simulink model "model6_yes"  (R2022a)
settings: Solver=FixedStepAuto  StartTime=0.0  StopTime=5  FixedStep=1e-5  RelTol=1e-3
model workspace (MAT data in the model file):
  b1 = 150
  b2 = 1500
  downSpringHeight = 10
  g = 9.81
  groundHeight = 100
  k1 = 7000
  k2 = 10000000
  m1 = 3.6
  m1IniHeight = 0
  m2 = 3.6
  m3 = 3.6
  upSpringHeight = 10
undefined symbols (not defined in the file or in its folder): DiscIntNeverNeededParam
settings Model: Creator=Tsing  LastModifiedBy=Tsing

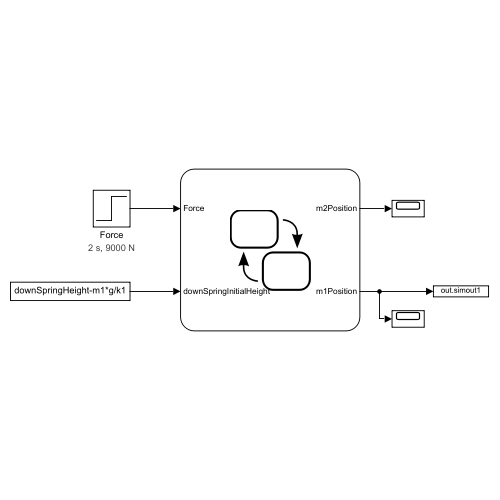
[thumbnail: Simulink's stored preview of the top-level diagram]
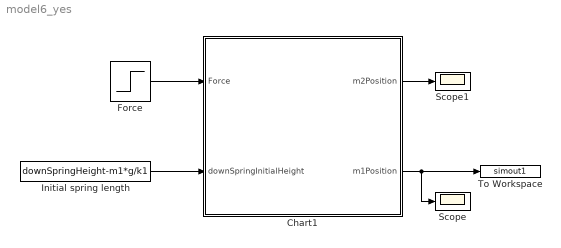
== system model6_yes ==
  Chart1 : Stateflow chart  TreatAsAtomicUnit=on
  Force : Step  Time=2  After=9000  SampleTime=0
      settings: AttributesFormatString=%<Time> s, %<After> N
  Initial spring length : Constant  Value=downSpringHeight-m1*g/k1
  Scope : Scope
  Scope1 : Scope
  To Workspace : ToWorkspace  VariableName=simout1  SaveFormat=Timeseries  SampleTime=-1
  wires:
  Force/1 -> Chart1/1(Force)
  Chart1/2(m1Position) -> To Workspace/1, Scope/1
  Initial spring length/1 -> Chart1/2(downSpringInitialHeight)
  Chart1/1(m2Position) -> Scope1/1

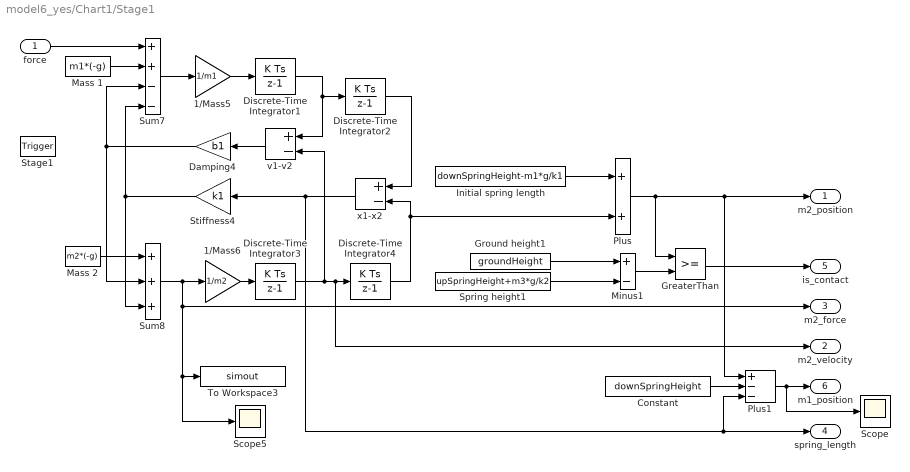
== system model6_yes/Chart1/Stage1 ==
  force : Inport  OutMin=1  OutMax=1  OutDataTypeStr=double  PortDimensions=1
  Stage1 : TriggerPort  TriggerType=function-call  VariantControl=(inherit)
      settings: CopyFcn=Stateflow.SLINSF.SimulinkMan.removeBlockPreDeleteFcn  PreDeleteFcn=Stateflow.SLINSF.SimulinkMan.unsafePredeleteFcn
  1/Mass5 : Gain  Gain=1/m1  SaturateOnIntegerOverflow=on  OutDataTypeStr=Inherit: Same as input  ParamDataTypeStr=Inherit: Same as input
  1/Mass6 : Gain  Gain=1/m2  SaturateOnIntegerOverflow=on  OutDataTypeStr=Inherit: Same as input  ParamDataTypeStr=Inherit: Same as input
  Constant : Constant  Value=downSpringHeight
  Damping4 : Gain  Gain=b1  SaturateOnIntegerOverflow=on  OutDataTypeStr=Inherit: Same as input  ParamDataTypeStr=Inherit: Same as input
  Discrete-Time Integrator1 : DiscreteIntegrator  InitialCondition=0.0  SampleTime=-1  ICPrevOutput=DiscIntNeverNeededParam  ICPrevScaledInput=DiscIntNeverNeededParam
  Discrete-Time Integrator2 : DiscreteIntegrator  InitialCondition=-m1*g/k1  SampleTime=-1  ICPrevOutput=DiscIntNeverNeededParam  ICPrevScaledInput=DiscIntNeverNeededParam
      settings: AttributesFormatString=x0 = %<InitialCondition> m
  Discrete-Time Integrator3 : DiscreteIntegrator  InitialCondition=0.0  SampleTime=-1  ICPrevOutput=DiscIntNeverNeededParam  ICPrevScaledInput=DiscIntNeverNeededParam
  Discrete-Time Integrator4 : DiscreteIntegrator  InitialCondition=0.0  SampleTime=-1  ICPrevOutput=DiscIntNeverNeededParam  ICPrevScaledInput=DiscIntNeverNeededParam
  GreaterThan : RelationalOperator  OutDataTypeStr=boolean  RndMeth=Simplest  InputSameDT=off
  Ground height1 : Constant  Value=groundHeight
  Initial spring length : Constant  Value=downSpringHeight-m1*g/k1
  Mass 1 : Constant  Value=m1*(-g)
  Mass 2 : Constant  Value=m2*(-g)
  Minus1 : Sum  Inputs=+-
  Plus : Sum
  Plus1 : Sum  Inputs=+--
  Scope : Scope
  Scope5 : Scope
  Spring height1 : Constant  Value=upSpringHeight+m3*g/k2
  Stiffness4 : Gain  Gain=k1  SaturateOnIntegerOverflow=on  OutDataTypeStr=Inherit: Same as input  ParamDataTypeStr=Inherit: Same as input
  Sum7 : Sum  Inputs=++--  InputSameDT=on  SaturateOnIntegerOverflow=on  OutDataTypeStr=Inherit: Same as first input
  Sum8 : Sum  Inputs=+++  InputSameDT=on  SaturateOnIntegerOverflow=on  OutDataTypeStr=Inherit: Same as first input
  To Workspace3 : ToWorkspace  VariableName=simout  SaveFormat=Timeseries  SampleTime=-1
  v1-v2 : Sum  Inputs=+-
  x1-x2 : Sum  Inputs=+-
  m2_position : Outport
  m2_velocity : Outport  Port=2
  m2_force : Outport  Port=3
  spring_length : Outport  Port=4
  is_contact : Outport  Port=5
  m1_position : Outport  Port=6
  wires:
  v1-v2/1 -> Damping4/1
  Sum8/1 -> Scope5/1, To Workspace3/1, m2_force/1, 1/Mass6/1
  Mass 2/1 -> Sum8/1
  force/1 -> Sum7/1
  Discrete-Time Integrator1/1 -> v1-v2/1, Discrete-Time Integrator2/1
  1/Mass6/1 -> Discrete-Time Integrator3/1
  Discrete-Time Integrator3/1 -> m2_velocity/1, Discrete-Time Integrator4/1, v1-v2/2
  Initial spring length/1 -> Plus/1
  Discrete-Time Integrator2/1 -> x1-x2/1
  Discrete-Time Integrator4/1 -> x1-x2/2, Plus/2
  x1-x2/1 -> Plus1/3, spring_length/1, Stiffness4/1
  Mass 1/1 -> Sum7/2
  1/Mass5/1 -> Discrete-Time Integrator1/1
  Plus/1 -> Plus1/1, m2_position/1, GreaterThan/1
  Stiffness4/1 -> Sum7/4, Sum8/3
  Sum7/1 -> 1/Mass5/1
  Damping4/1 -> Sum7/3, Sum8/2
  Ground height1/1 -> Minus1/1
  Spring height1/1 -> Minus1/2
  Minus1/1 -> GreaterThan/2
  GreaterThan/1 -> is_contact/1
  Plus1/1 -> Scope/1, m1_position/1
  Constant/1 -> Plus1/2

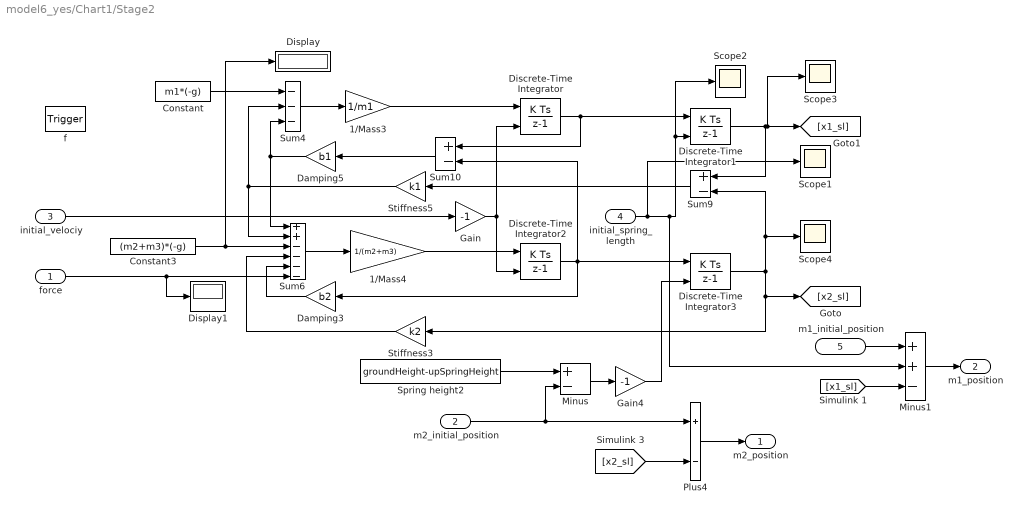
== system model6_yes/Chart1/Stage2 ==
  force : Inport  OutMin=1  OutMax=1  OutDataTypeStr=double  PortDimensions=1
  m2_initial_position : Inport  Port=2  OutMin=1  OutMax=1  OutDataTypeStr=double  PortDimensions=1
  initial_velociy : Inport  Port=3  OutMin=1  OutMax=1  OutDataTypeStr=double  PortDimensions=1
  initial_spring_length : Inport  Port=4  OutMin=1  OutMax=1  OutDataTypeStr=double  PortDimensions=1
  m1_initial_position : Inport  Port=5  OutMin=1  OutMax=1  OutDataTypeStr=double  PortDimensions=1
  f : TriggerPort  TriggerType=function-call  VariantControl=(inherit)
      settings: CopyFcn=Stateflow.SLINSF.SimulinkMan.removeBlockPreDeleteFcn  PreDeleteFcn=Stateflow.SLINSF.SimulinkMan.unsafePredeleteFcn
  1/Mass3 : Gain  Gain=1/m1  SaturateOnIntegerOverflow=on  OutDataTypeStr=Inherit: Same as input  ParamDataTypeStr=Inherit: Same as input
  1/Mass4 : Gain  Gain=1/(m2+m3)  SaturateOnIntegerOverflow=on  OutDataTypeStr=Inherit: Same as input  ParamDataTypeStr=Inherit: Same as input
  Constant : Constant  Value=m1*(-g)  SampleTime=-1
  Constant3 : Constant  Value=(m2+m3)*(-g)  SampleTime=-1
  Damping3 : Gain  Gain=b2  SaturateOnIntegerOverflow=on  OutDataTypeStr=Inherit: Same as input  ParamDataTypeStr=Inherit: Same as input
  Damping5 : Gain  Gain=b1  SaturateOnIntegerOverflow=on  OutDataTypeStr=Inherit: Same as input  ParamDataTypeStr=Inherit: Same as input
  Discrete-Time Integrator{,1..3} (4 alike) : DiscreteIntegrator  InitialConditionSource=external  SampleTime=-1  ICPrevOutput=DiscIntNeverNeededParam  ICPrevScaledInput=DiscIntNeverNeededParam
  Display : Display
  Display1 : Display
  Gain : Gain  Gain=-1
  Gain4 : Gain  Gain=-1
  Minus : Sum  Inputs=+-
  Minus1 : Sum  Inputs=++-
  Plus4 : Sum  Inputs=+-
  Scope{1..4} (4 alike) : Scope
  Spring height2 : Constant  Value=groundHeight-upSpringHeight  SampleTime=-1
  Stiffness3 : Gain  Gain=k2  SaturateOnIntegerOverflow=on  OutDataTypeStr=Inherit: Same as input  ParamDataTypeStr=Inherit: Same as input
  Stiffness5 : Gain  Gain=k1  SaturateOnIntegerOverflow=on  OutDataTypeStr=Inherit: Same as input  ParamDataTypeStr=Inherit: Same as input
  Sum10 : Sum  Inputs=+-  InputSameDT=on  SaturateOnIntegerOverflow=on  OutDataTypeStr=Inherit: Same as first input
  Sum4 : Sum  Inputs=---  InputSameDT=on  SaturateOnIntegerOverflow=on  OutDataTypeStr=Inherit: Same as first input
  Sum6 : Sum  Inputs=++----  InputSameDT=on  SaturateOnIntegerOverflow=on  OutDataTypeStr=Inherit: Same as first input
  Sum9 : Sum  Inputs=+-  InputSameDT=on  SaturateOnIntegerOverflow=on  OutDataTypeStr=Inherit: Same as first input
  m2_position : Outport
  m1_position : Outport  Port=2
  wires:
  Constant/1 -> Sum4/1
  Discrete-Time Integrator3/1 -> Scope4/1, Sum9/2, Stiffness3/1, [x2_sl]
  Damping3/1 -> Sum6/5
  Gain4/1 -> Discrete-Time Integrator3/2
  Sum4/1 -> 1/Mass3/1
  Sum6/1 -> 1/Mass4/1
  Gain/1 -> Discrete-Time Integrator2/2, Discrete-Time Integrator/2
  Plus4/1 -> m2_position/1
  m2_initial_position/1 -> Minus/2, Plus4/1
  Sum9/1 -> Stiffness5/1
  Stiffness5/1 -> Sum6/2, Sum4/2
  1/Mass4/1 -> Discrete-Time Integrator2/1
  Discrete-Time Integrator2/1 -> Sum10/2, Discrete-Time Integrator3/1, Damping3/1
  [x2_sl] -> Plus4/2
  Stiffness3/1 -> Sum6/4
  Damping5/1 -> Sum4/3, Sum6/1
  force/1 -> Sum6/6, Display1/1
  Constant3/1 -> Display/1, Sum6/3
  initial_velociy/1 -> Gain/1
  Sum10/1 -> Damping5/1
  Discrete-Time Integrator/1 -> Discrete-Time Integrator1/1, Sum10/1
  Discrete-Time Integrator1/1 -> Scope3/1, [x1_sl], Sum9/1
  1/Mass3/1 -> Discrete-Time Integrator/1
  Minus/1 -> Gain4/1
  Spring height2/1 -> Minus/1
  initial_spring_length/1 -> Scope1/1, Minus1/2, Scope2/1, Discrete-Time Integrator1/2
  Minus1/1 -> m1_position/1
  m1_initial_position/1 -> Minus1/1
  [x1_sl] -> Minus1/3

== stateflow chart model6_yes/Chart1 ==
  state BeginStage2
    [m2_position_stage2,m1_position_stage2] = ...
    Stage2(m2_force_stage1,m2_position_stage1,m2_velocity_stage1,spring_length_stage1,m1_position_stage1);
    m2Position = m2_position_stage2;
    m1Position = m1_position_stage2;
  state BeginStage1
    [m2_position_stage1,m2_velocity_stage1, ...
    m2_force_stage1,spring_length_stage1,is_contact,m1_position_stage1] = Stage1(Force);
    m2Position = m2_position_stage1;
    m1Position = m1_position_stage1;
  state Still
    m2Position = downSpringInitialHeight;
    m1Position = 0;
  state [m2_position,m2_velocity,m2_force,spring_length,is_contact,m1_position] = Stage1(force) [function]
  state [m2_position,m1_position] = Stage2(force,m2_initial_position,initial_velociy,initial_spring_length,m1_initial_position) [function]
  (default) -> Still
  BeginStage1 -> BeginStage2 : [is_contact == 1]
  Still -> BeginStage1 : [Force > 0]
  data: force function_input double size=1; m2_position function_output; m2_velocity function_output; m2_force function_output; spring_length function_output; is_contact function_output; m1_position function_output; force function_input double size=1; m2_initial_position function_input double size=1; initial_velociy function_input double size=1; initial_spring_length function_input double size=1; m2_position function_output; m1_position function_output; m1_initial_position function_input double size=1; Force input; downSpringInitialHeight input; m2Position output size=1; m1Position output size=1; is_contact local; m1_position_stage1 local; m2_force_stage1 local; m2_position_stage1 local; m2_velocity_stage1 local; spring_length_stage1 local; m1_position_stage2 local; m2_position_stage2 local
